simulink model "motor_model2"  (R2021a)
settings: Solver=FixedStepAuto  StartTime=0.0  StopTime=10.0  FixedStep=25e-6  RelTol=1e-3
values from neighbouring files (symbols this model uses):
  B = 0.01    [data_motor2.m]
  kePhi = 1.6    [data_motor2.m]
  Ra = 0.5    [data_motor2.m]
  tau_a = La/Ra    (= 0.2)    [data_motor2.m]
  tau_m = J/B    (= 500)    [data_motor2.m]
  TL = 20    [data_motor2.m]
  Va = 160    [data_motor2.m]
libraries: simulink_extras x2, spspowerguiLib x1
settings Model: Creator=Davie  LastModifiedBy=Davie

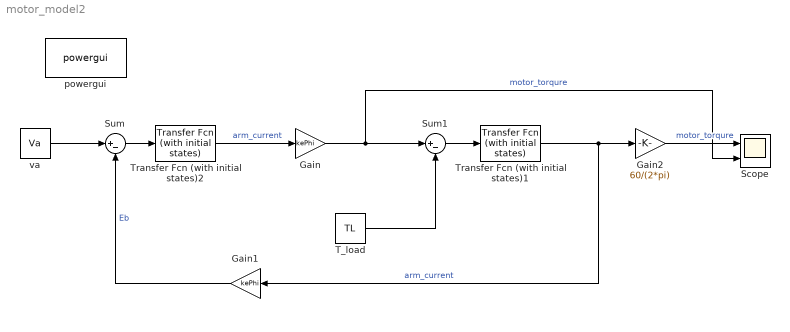
== system motor_model2 ==
  Gain : Gain  Gain=kePhi
  Gain1 : Gain  Gain=kePhi
  Gain2 : Gain  Gain=60/(2*pi)
  Scope : Scope  NumInputPorts=2
  Sum : Sum  Inputs=|+-
  Sum1 : Sum  Inputs=|+-
  T_load : Constant  Value=TL
  Transfer Fcn (with initial states)1 : simulink_extras/Additional Linear/Transfer Fcn (with initial states)  N=[1/B]  D=[tau_m 1 ]  X0=0
  Transfer Fcn (with initial states)2 : simulink_extras/Additional Linear/Transfer Fcn (with initial states)  N=[1/Ra]  D=[tau_a 1 ]  X0=0
  powergui : spspowerguiLib/powergui  Priority=1  SimulationMode=Continuous  SampleTime=50e-6  frequency=60  Iterations=50  frequencyindice=60  Pbase=100e6  ErrMax=1e-4  UnitsV=kV  UnitsW=MW  buscounter=0  FunctionMessages=off  echomessages=off  EnableUseOfTLC=off  CurrentSourceSwitches=off  DisableSnubberDevices=off  DisableRonSwitches=off  DisableVfSwitches=off  DisplayEquations=off  AutomaticDiscreteSolvers=off  SolverType=Tustin/Backward Euler (TBE)  Interpol=off  ExternalGateDelay=off  methode=off  Ts=100  x0status=blocks  SPID=on  SwTol=0  HookPort=off  NonlinearTolerance=1e-4  nMaxIteration=100  ContinueOnMaxIteration=off  RestoreLinks=warning  ResistiveCurrentMeasurement=off  Frange=[0:2:500]  Ylog=off  Xlog=on  ShowGrid=off  save=off  variable=ZData  structure=0  ZoomFFT=off  StartTime=0.0  cycles=1  DisplayStyle=1  fundamental=60  FreqAxis=off  MaxFrequency=1000  frequencyindicesteady=1  RmsSteady=1  display=off
  "va " : Constant  Value=Va
  wires:
  "va "/1 -> Sum/1
  Sum/1 -> Transfer Fcn (with initial states)2/1
  Transfer Fcn (with initial states)2/1 -> Gain/1  "arm_current"
  Gain/1 -> Scope/2, Sum1/1  "motor_torqure"
  T_load/1 -> Sum1/2
  Sum1/1 -> Transfer Fcn (with initial states)1/1
  Transfer Fcn (with initial states)1/1 -> Gain1/1, Gain2/1  "arm_current"
  Gain1/1 -> Sum/2  "Eb"
  Gain2/1 -> Scope/1  "motor_torqure"
